simulink model "Gewerk2_Bahnplanung2015"  (Simulink 8.6)
settings: Solver=ode3  StartTime=0.0  StopTime=inf  FixedStep=0.005  RelTol=1e-3
undefined symbols (not defined in the file or in its folder): Com1, none
libraries: xpcrtudplib x9, xpcutilitieslib x5, xpcseriallib x1, slrtlib x1
(part 2 of 2)

== matlab function Gewerk2/Globale Markierung ==
  data: Robbi input double; StationArray input double; FifoArray input double; FifoArray1 output double; StationArray1 output double
function [FifoArray1,StationArray1]= fcn(Robbi,StationArray,FifoArray)
%#codegen
X=[Robbi(1) Robbi(4) Robbi(7) Robbi(10)];
Y=[Robbi(2) Robbi(5) Robbi(8) Robbi(11)];
FifoArray1=zeroes([1 12]);
FifoArray1=FifoArray;
StationArray1=zeroes([1 8]);
StationArray1=StationArray;
N=zeroes([1 12]);
S=Zeroes([1 8]);
for n= 1 : 1 : 4
    N(n)=round((X(n)-528)/400);   % Berechnung in welchem Fifo der Roboter sich befindet
    S(n)=round((X(n)-725)/560);   %Berechnung in welcher Station der Roboter sich befindet
    if (Y(n)<=2100 || Y(n)>3400)
        for i=1:8
            if StationArray1(i)==n
                StationArray(i)=0;
            end
        end
    end
    if (Y(n)>2100 && X(n)<5100) 
         for i=1:12
            if FifoArray1(i)==n
                FifoArray1(i)=0;
            end
        end
        StationArray1(S(n))=n;
        
    else if (Y(n)<450 && (X(n)>100 && X(n)<5250))
        for i=1:12
            if FifoArray1(i)==n
                FifoArray1(i)=0;
            end
        end
            FifoArray1(N(n))=n;
        end
    end
end
